simulink model "GradingSystem"  (R2017b)
settings: Solver=FixedStepDiscrete  StartTime=0.0  StopTime=10.0  RelTol=1e-3
settings Model: Creator=engdo  LastModifiedBy=engdo
settings OptimizationCC: DefaultParameterBehavior=Inlined  PassReuseOutputArgsAs=Individual arguments
settings DebuggingCC: ParameterTunabilityLossMsg=error
settings SFSimCC: MATLABDynamicMemAlloc=off
settings RTWCC: SystemTargetFile=ert.tlc  GenCodeOnly=on  TemplateMakefile=ert_default_tmf  GenerateReport=on  IncludeHyperlinkInReport=on  LaunchReport=on  GenerateTraceInfo=on  GenerateTraceReport=on  GenerateTraceReportSl=on  GenerateTraceReportSf=on  GenerateTraceReportEml=on  GenerateWebview=on
settings CodeAppCC: ForceParamTrailComments=on  IgnoreCustomStorageClasses=off  OperatorAnnotations=on  SimulinkDataObjDesc=on  SFDataObjDesc=on  InsertBlockDesc=on
settings ERTTargetCC: TargetLangStandard=C99 (ISO)  GenerateSampleERTMain=on  InlinedParameterPlacement=NonHierarchical  ERTCustomFileTemplate=example_file_process.tlc  EnableUserReplacementTypes=on

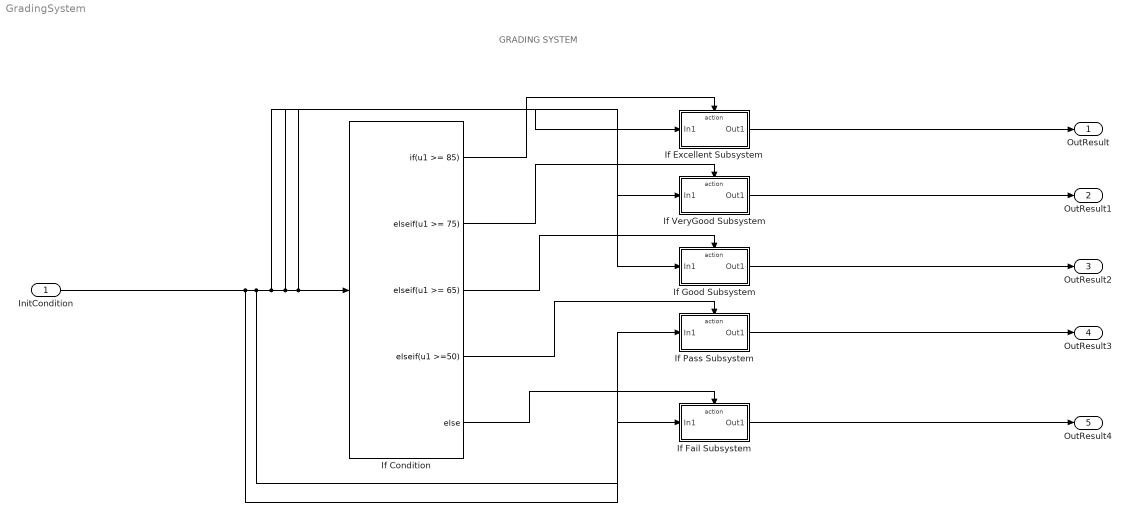
== system GradingSystem ==
  note: GRADING SYSTEM
  InitCondition : Inport
  If Condition : If  IfExpression=u1 >= 85  ElseIfExpressions=u1 >= 75,u1 >= 65,u1 >=50
  If Excellent Subsystem : Subsystem  TreatAsAtomicUnit=on
  If Fail Subsystem : Subsystem  TreatAsAtomicUnit=on
  If Good Subsystem : Subsystem  TreatAsAtomicUnit=on
  If Pass Subsystem : Subsystem  TreatAsAtomicUnit=on
  If VeryGood Subsystem : Subsystem  TreatAsAtomicUnit=on
  OutResult : Outport
  OutResult1 : Outport  Port=2
  OutResult2 : Outport  Port=3
  OutResult3 : Outport  Port=4
  OutResult4 : Outport  Port=5
  wires:
  If Condition/1 -> If Excellent Subsystem/Action
  If Condition/2 -> If VeryGood Subsystem/Action
  If Condition/3 -> If Good Subsystem/Action
  If Condition/4 -> If Pass Subsystem/Action
  If Condition/5 -> If Fail Subsystem/Action
  If Fail Subsystem/1(Out1) -> OutResult4/1
  If Pass Subsystem/1(Out1) -> OutResult3/1
  If Good Subsystem/1(Out1) -> OutResult2/1
  If VeryGood Subsystem/1(Out1) -> OutResult1/1
  InitCondition/1 -> If Fail Subsystem/1(In1), If Pass Subsystem/1(In1), If Good Subsystem/1(In1), If VeryGood Subsystem/1(In1), If Excellent Subsystem/1(In1), If Condition/1
  If Excellent Subsystem/1(Out1) -> OutResult/1

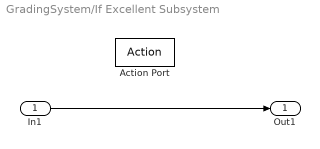
== system GradingSystem/If Excellent Subsystem ==
  In1 : Inport
  Action Port : ActionPort  ActionType=then
  Out1 : Outport
  wires:
  In1/1 -> Out1/1

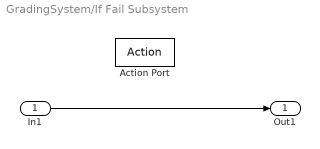
== system GradingSystem/If Fail Subsystem ==
  In1 : Inport
  Action Port : ActionPort  ActionType=else
  Out1 : Outport
  wires:
  In1/1 -> Out1/1

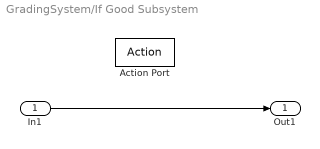
== system GradingSystem/If Good Subsystem ==
  In1 : Inport
  Action Port : ActionPort  ActionType=elseif
  Out1 : Outport
  wires:
  In1/1 -> Out1/1

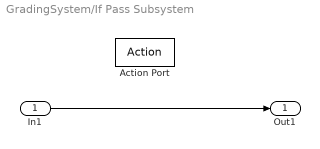
== system GradingSystem/If Pass Subsystem ==
  In1 : Inport
  Action Port : ActionPort  ActionType=elseif
  Out1 : Outport
  wires:
  In1/1 -> Out1/1

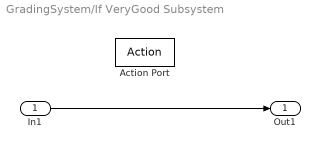
== system GradingSystem/If VeryGood Subsystem ==
  In1 : Inport
  Action Port : ActionPort  ActionType=elseif
  Out1 : Outport
  wires:
  In1/1 -> Out1/1
